simulink model "Model_Platform"  (R2018a)
settings: Solver=ode1  StartTime=0.0  StopTime=inf  FixedStep=0.001  RelTol=1e-3  EnableMultiTasking=on
PreLoadFcn:
  | ;HLABlocksetInit;;HLABlocksetInit;;HLABlocksetInit;
PostLoadFcn:
  | ;set_param(gcs,'PostCodeGenCommand', 'rtw_defines(buildInfo)');;set_param(gcs,'PostCodeGenCommand', 'rtw_defines(buildInfo)');;set_param(gcs,'PostCodeGenCommand', 'rtw_defines(buildInfo)');
undefined symbols (not defined in the file or in its folder): eng_speed, Heading_init, inertiaLateral, Joystick, Newton, omega_engine, omega_max, omega_wheel, Para, radiusWheel, Raphson, Standard_Devices, torque, Torque_lost, Torque_lost_wheel, X_init, Y_init, Z_init
libraries: simulink x26, dspnetwork x4, rtwinlib x2, PC_Simulator_Lib x2, vrlib x1
(part 4 of 4)

== system Model_Platform/Vehicle model/Drive_Train/4_Wheels_drive_train_and_Brake/FL/Alpha_Kappa_Selector2/alpha_calc/front ==
  Vy : Inport
  Vx : Inport  Port=2
  steering_angle : Inport  Port=3
  Constant : Constant  Value=0.001
  Divide : Product  Inputs=*/
  Fcn : Fcn  Expr=atan(u)
  Gain : Gain  Gain=180/pi
  Relational Operator : RelationalOperator  OutDataTypeStr=boolean  RndMeth=Nearest
  Subsystem1 : Subsystem
  Subtract : Sum  Inputs=+-
  Switch : Switch  Threshold=1
  alpha : Outport
  wires:
  Subsystem1/1(Out1) -> Divide/1
  Vx/1 -> Switch/1, Relational Operator/1
  Vy/1 -> Subsystem1/1(In1)
  Switch/1 -> Divide/2
  Fcn/1 -> Subtract/2
  Gain/1 -> alpha/1
  Divide/1 -> Fcn/1
  Subtract/1 -> Gain/1
  steering_angle/1 -> Subtract/1
  Constant/1 -> Relational Operator/2, Switch/3
  Relational Operator/1 -> Switch/2

== system Model_Platform/Vehicle model/Drive_Train/4_Wheels_drive_train_and_Brake/FR/Alpha_Kappa_Selector2/Dynamik Anteil2/Subsystem3 ==
  In1 : Inport
  Abs : Abs  SaturateOnIntegerOverflow=on
  In3_Switch : Constant
  Relational Operator : RelationalOperator  RndMeth=Nearest
  Switch : Switch  Threshold=1  SaturateOnIntegerOverflow=on
  Out1 : Outport
  wires:
  Switch/1 -> Out1/1
  Relational Operator/1 -> Switch/2
  In3_Switch/1 -> Switch/3, Relational Operator/2
  Abs/1 -> Relational Operator/1
  In1/1 -> Abs/1, Switch/1

== system Model_Platform/Vehicle model/Drive_Train/4_Wheels_drive_train_and_Brake/FR/Alpha_Kappa_Selector2/alpha_calc/Slip_angle_Calculation_From_Vx_and_Vy1 ==
  Vx_CoG[m|s] : Inport
  Vy_CoG[m|s] : Inport  Port=2
  Add : Sum
  Add2 : Sum
  Compare To Constant1 : simulink/Logic and Bit Operations/Compare To Constant  relop=>=  const=1  OutDataTypeStr=boolean
  Constant1 : Constant  Value=eps
  Data Type Conversion : DataTypeConversion
  Divide : Product  Inputs=*/
  Gain : Gain  Gain=180/pi
  Math Function : Math  Operator=square  SaturateOnIntegerOverflow=on
  Math Function1 : Math  Operator=square  SaturateOnIntegerOverflow=on
  Product1 : Product  Inputs=3
  Sign : Signum
  Sqrt : Sqrt  AlgorithmType=Newton-Raphson  SaturateOnIntegerOverflow=on
  Trigonometric Function1 : Trigonometry  Operator=atan
  Unary Minus1 : UnaryMinus
  Slip_Angle[deg] : Outport
  wires:
  Unary Minus1/1 -> Product1/3
  Sign/1 -> Unary Minus1/1
  Trigonometric Function1/1 -> Product1/1
  Constant1/1 -> Add2/2
  Add2/1 -> Divide/2
  Divide/1 -> Trigonometric Function1/1
  Sqrt/1 -> Compare To Constant1/1
  Add/1 -> Sqrt/1
  Math Function1/1 -> Add/2
  Math Function/1 -> Add/1
  Vx_CoG[m|s]/1 -> Add2/1, Math Function/1, Sign/1
  Vy_CoG[m|s]/1 -> Divide/1, Math Function1/1
  Compare To Constant1/1 -> Data Type Conversion/1
  Data Type Conversion/1 -> Product1/2
  Product1/1 -> Gain/1
  Gain/1 -> Slip_Angle[deg]/1

== system Model_Platform/Vehicle model/Drive_Train/4_Wheels_drive_train_and_Brake/FR/Alpha_Kappa_Selector2/alpha_calc/front ==
  Vy : Inport
  Vx : Inport  Port=2
  steering_angle : Inport  Port=3
  Constant : Constant  Value=0.001
  Divide : Product  Inputs=*/
  Fcn : Fcn  Expr=atan(u)
  Gain : Gain  Gain=180/pi
  Relational Operator : RelationalOperator  OutDataTypeStr=boolean  RndMeth=Nearest
  Subsystem1 : Subsystem
  Subtract : Sum  Inputs=+-
  Switch : Switch  Threshold=1
  alpha : Outport
  wires:
  Subsystem1/1(Out1) -> Divide/1
  Vx/1 -> Switch/1, Relational Operator/1
  Vy/1 -> Subsystem1/1(In1)
  Switch/1 -> Divide/2
  Fcn/1 -> Subtract/2
  Gain/1 -> alpha/1
  Divide/1 -> Fcn/1
  Subtract/1 -> Gain/1
  steering_angle/1 -> Subtract/1
  Constant/1 -> Relational Operator/2, Switch/3
  Relational Operator/1 -> Switch/2

== system Model_Platform/Vehicle model/Drive_Train/4_Wheels_drive_train_and_Brake/RL/Alpha_Kappa_Selector2/Dynamik Anteil2/Subsystem3 ==
  In1 : Inport
  Abs : Abs  SaturateOnIntegerOverflow=on
  In3_Switch : Constant
  Relational Operator : RelationalOperator  RndMeth=Nearest
  Switch : Switch  Threshold=1  SaturateOnIntegerOverflow=on
  Out1 : Outport
  wires:
  Switch/1 -> Out1/1
  Relational Operator/1 -> Switch/2
  In3_Switch/1 -> Switch/3, Relational Operator/2
  Abs/1 -> Relational Operator/1
  In1/1 -> Abs/1, Switch/1

== system Model_Platform/Vehicle model/Drive_Train/4_Wheels_drive_train_and_Brake/RL/Alpha_Kappa_Selector2/alpha_calc/Slip_angle_Calculation_From_Vx_and_Vy1 ==
  Vx_CoG[m|s] : Inport
  Vy_CoG[m|s] : Inport  Port=2
  Add : Sum
  Add2 : Sum
  Compare To Constant1 : simulink/Logic and Bit Operations/Compare To Constant  relop=>=  const=1  OutDataTypeStr=boolean
  Constant1 : Constant  Value=eps
  Data Type Conversion : DataTypeConversion
  Divide : Product  Inputs=*/
  Gain : Gain  Gain=180/pi
  Math Function : Math  Operator=square  SaturateOnIntegerOverflow=on
  Math Function1 : Math  Operator=square  SaturateOnIntegerOverflow=on
  Product1 : Product  Inputs=3
  Sign : Signum
  Sqrt : Sqrt  AlgorithmType=Newton-Raphson  SaturateOnIntegerOverflow=on
  Trigonometric Function1 : Trigonometry  Operator=atan
  Unary Minus1 : UnaryMinus
  Slip_Angle[deg] : Outport
  wires:
  Unary Minus1/1 -> Product1/3
  Sign/1 -> Unary Minus1/1
  Trigonometric Function1/1 -> Product1/1
  Constant1/1 -> Add2/2
  Add2/1 -> Divide/2
  Divide/1 -> Trigonometric Function1/1
  Sqrt/1 -> Compare To Constant1/1
  Add/1 -> Sqrt/1
  Math Function1/1 -> Add/2
  Math Function/1 -> Add/1
  Vx_CoG[m|s]/1 -> Add2/1, Math Function/1, Sign/1
  Vy_CoG[m|s]/1 -> Divide/1, Math Function1/1
  Compare To Constant1/1 -> Data Type Conversion/1
  Data Type Conversion/1 -> Product1/2
  Product1/1 -> Gain/1
  Gain/1 -> Slip_Angle[deg]/1

== system Model_Platform/Vehicle model/Drive_Train/4_Wheels_drive_train_and_Brake/RL/Alpha_Kappa_Selector2/alpha_calc/front ==
  Vy : Inport
  Vx : Inport  Port=2
  steering_angle : Inport  Port=3
  Constant : Constant  Value=0.001
  Divide : Product  Inputs=*/
  Fcn : Fcn  Expr=atan(u)
  Gain : Gain  Gain=180/pi
  Relational Operator : RelationalOperator  OutDataTypeStr=boolean  RndMeth=Nearest
  Subsystem1 : Subsystem
  Subtract : Sum  Inputs=+-
  Switch : Switch  Threshold=1
  alpha : Outport
  wires:
  Subsystem1/1(Out1) -> Divide/1
  Vx/1 -> Switch/1, Relational Operator/1
  Vy/1 -> Subsystem1/1(In1)
  Switch/1 -> Divide/2
  Fcn/1 -> Subtract/2
  Gain/1 -> alpha/1
  Divide/1 -> Fcn/1
  Subtract/1 -> Gain/1
  steering_angle/1 -> Subtract/1
  Constant/1 -> Relational Operator/2, Switch/3
  Relational Operator/1 -> Switch/2

== system Model_Platform/Vehicle model/Drive_Train/4_Wheels_drive_train_and_Brake/RR/Alpha_Kappa_Selector2/Dynamik Anteil2/Subsystem3 ==
  In1 : Inport
  Abs : Abs  SaturateOnIntegerOverflow=on
  In3_Switch : Constant
  Relational Operator : RelationalOperator  RndMeth=Nearest
  Switch : Switch  Threshold=1  SaturateOnIntegerOverflow=on
  Out1 : Outport
  wires:
  Switch/1 -> Out1/1
  Relational Operator/1 -> Switch/2
  In3_Switch/1 -> Switch/3, Relational Operator/2
  Abs/1 -> Relational Operator/1
  In1/1 -> Abs/1, Switch/1

== system Model_Platform/Vehicle model/Drive_Train/4_Wheels_drive_train_and_Brake/RR/Alpha_Kappa_Selector2/alpha_calc/Slip_angle_Calculation_From_Vx_and_Vy1 ==
  Vx_CoG[m|s] : Inport
  Vy_CoG[m|s] : Inport  Port=2
  Add : Sum
  Add2 : Sum
  Compare To Constant1 : simulink/Logic and Bit Operations/Compare To Constant  relop=>=  const=1  OutDataTypeStr=boolean
  Constant1 : Constant  Value=eps
  Data Type Conversion : DataTypeConversion
  Divide : Product  Inputs=*/
  Gain : Gain  Gain=180/pi
  Math Function : Math  Operator=square  SaturateOnIntegerOverflow=on
  Math Function1 : Math  Operator=square  SaturateOnIntegerOverflow=on
  Product1 : Product  Inputs=3
  Sign : Signum
  Sqrt : Sqrt  AlgorithmType=Newton-Raphson  SaturateOnIntegerOverflow=on
  Trigonometric Function1 : Trigonometry  Operator=atan
  Unary Minus1 : UnaryMinus
  Slip_Angle[deg] : Outport
  wires:
  Unary Minus1/1 -> Product1/3
  Sign/1 -> Unary Minus1/1
  Trigonometric Function1/1 -> Product1/1
  Constant1/1 -> Add2/2
  Add2/1 -> Divide/2
  Divide/1 -> Trigonometric Function1/1
  Sqrt/1 -> Compare To Constant1/1
  Add/1 -> Sqrt/1
  Math Function1/1 -> Add/2
  Math Function/1 -> Add/1
  Vx_CoG[m|s]/1 -> Add2/1, Math Function/1, Sign/1
  Vy_CoG[m|s]/1 -> Divide/1, Math Function1/1
  Compare To Constant1/1 -> Data Type Conversion/1
  Data Type Conversion/1 -> Product1/2
  Product1/1 -> Gain/1
  Gain/1 -> Slip_Angle[deg]/1

== system Model_Platform/Vehicle model/Drive_Train/4_Wheels_drive_train_and_Brake/RR/Alpha_Kappa_Selector2/alpha_calc/front ==
  Vy : Inport
  Vx : Inport  Port=2
  steering_angle : Inport  Port=3
  Constant : Constant  Value=0.001
  Divide : Product  Inputs=*/
  Fcn : Fcn  Expr=atan(u)
  Gain : Gain  Gain=180/pi
  Relational Operator : RelationalOperator  OutDataTypeStr=boolean  RndMeth=Nearest
  Subsystem1 : Subsystem
  Subtract : Sum  Inputs=+-
  Switch : Switch  Threshold=1
  alpha : Outport
  wires:
  Subsystem1/1(Out1) -> Divide/1
  Vx/1 -> Switch/1, Relational Operator/1
  Vy/1 -> Subsystem1/1(In1)
  Switch/1 -> Divide/2
  Fcn/1 -> Subtract/2
  Gain/1 -> alpha/1
  Divide/1 -> Fcn/1
  Subtract/1 -> Gain/1
  steering_angle/1 -> Subtract/1
  Constant/1 -> Relational Operator/2, Switch/3
  Relational Operator/1 -> Switch/2

== system Model_Platform/Vehicle model/Drive_Train/4_Wheels_drive_train_and_Brake/FL/Alpha_Kappa_Selector2/alpha_calc/front/Subsystem1 ==
  In1 : Inport
  Abs : Abs
  Constant1 : Constant  Value=0.005
  Constant2 : Constant  Value=0
  Relational Operator1 : RelationalOperator  OutDataTypeStr=boolean  RndMeth=Nearest
  Switch1 : Switch  Threshold=1
  Out1 : Outport
  wires:
  In1/1 -> Switch1/1, Abs/1
  Relational Operator1/1 -> Switch1/2
  Switch1/1 -> Out1/1
  Constant1/1 -> Relational Operator1/2
  Constant2/1 -> Switch1/3
  Abs/1 -> Relational Operator1/1

== system Model_Platform/Vehicle model/Drive_Train/4_Wheels_drive_train_and_Brake/FR/Alpha_Kappa_Selector2/alpha_calc/front/Subsystem1 ==
  In1 : Inport
  Abs : Abs
  Constant1 : Constant  Value=0.005
  Constant2 : Constant  Value=0
  Relational Operator1 : RelationalOperator  OutDataTypeStr=boolean  RndMeth=Nearest
  Switch1 : Switch  Threshold=1
  Out1 : Outport
  wires:
  In1/1 -> Switch1/1, Abs/1
  Relational Operator1/1 -> Switch1/2
  Switch1/1 -> Out1/1
  Constant1/1 -> Relational Operator1/2
  Constant2/1 -> Switch1/3
  Abs/1 -> Relational Operator1/1

== system Model_Platform/Vehicle model/Drive_Train/4_Wheels_drive_train_and_Brake/RL/Alpha_Kappa_Selector2/alpha_calc/front/Subsystem1 ==
  In1 : Inport
  Abs : Abs
  Constant1 : Constant  Value=0.005
  Constant2 : Constant  Value=0
  Relational Operator1 : RelationalOperator  OutDataTypeStr=boolean  RndMeth=Nearest
  Switch1 : Switch  Threshold=1
  Out1 : Outport
  wires:
  In1/1 -> Switch1/1, Abs/1
  Relational Operator1/1 -> Switch1/2
  Switch1/1 -> Out1/1
  Constant1/1 -> Relational Operator1/2
  Constant2/1 -> Switch1/3
  Abs/1 -> Relational Operator1/1

== system Model_Platform/Vehicle model/Drive_Train/4_Wheels_drive_train_and_Brake/RR/Alpha_Kappa_Selector2/alpha_calc/front/Subsystem1 ==
  In1 : Inport
  Abs : Abs
  Constant1 : Constant  Value=0.005
  Constant2 : Constant  Value=0
  Relational Operator1 : RelationalOperator  OutDataTypeStr=boolean  RndMeth=Nearest
  Switch1 : Switch  Threshold=1
  Out1 : Outport
  wires:
  In1/1 -> Switch1/1, Abs/1
  Relational Operator1/1 -> Switch1/2
  Switch1/1 -> Out1/1
  Constant1/1 -> Relational Operator1/2
  Constant2/1 -> Switch1/3
  Abs/1 -> Relational Operator1/1

== matlab function Model_Platform/Vehicle model/Drive_Train/4_Wheels_drive_train_and_Brake/FL/Fx_calculator ==
  data: lambda input; Fx output; alpha input; Fz input; mue input
 function Fx = FM_Fx(lambda,alpha,Fz,mue)
% This block supports an embeddable subset of the MATLAB language.
% See the help menu for details. 

%% Längstkraft
kappa=lambda;
a=tan(alpha*pi/180);
F_z=Fz;
% Parameter
p_Cx1=1.685;
p_Ex1=0.344;
p_Ex2=0.095;
p_Ex3=-0.02;
p_Ex4=0;
p_Kx1=21.51;
p_Kx2=-0.163;
p_Kx3=0.245;
p_Hx1=0;
p_Hx2=0;
p_Vx1=0;
p_Vx2=0;
r_Cx1=1.0902;
r_Bx1=12.35;
r_Bx2=-10.77;
r_Bx3=0;
r_Ex1=0;
r_Ex2=0;
r_Hx1=0.007;            %r_Hx1=0.007;
gamma=0;
lambda_xa=1;
lambda_Cx=1;
lambda_Ex=1;
lambda_Hx=1;
lambda_Vx=1;
lambda_Kxkappa=1;
% Unter der Annahme, dass die Vertikallast unverändert bleibt:
df_z=0;

%F_z=5500;
%mue=0.7;
chi_1=1;

% Berechnung:

B_xa=(r_Bx1+r_Bx3*gamma^2)*cos(atan(r_Bx2*kappa))*lambda_xa;
C_xa=r_Cx1;
E_xa=r_Ex1+r_Ex2*df_z;

S_Hxa=r_Hx1;
a_S=a+S_Hxa;

G_xa0=cos(C_xa*atan(B_xa*S_Hxa-E_xa*(B_xa*S_Hxa-atan(B_xa*S_Hxa))));
G_xa=cos(C_xa*atan(B_xa*a_S-E_xa*(B_xa*a_S-atan(B_xa*a_S))))/G_xa0;

K_xkappa=F_z*(p_Kx1+p_Kx2*df_z)*exp(p_Kx3*df_z)*lambda_Kxkappa;
C_x=p_Cx1*lambda_Cx;
D_x=mue*F_z*chi_1;
B_x=K_xkappa/(C_x*D_x+eps);
E_x=(p_Ex1+p_Ex2*df_z+p_Ex3*df_z^2)*(1-p_Ex4*sign(kappa))*lambda_Ex;

S_Vx=F_z*(p_Vx1+p_Vx2*df_z)*lambda_Vx*lambda_Hx*chi_1;
S_Hx=(p_Hx1+p_Hx2*df_z)*lambda_Hx;
kappa_x=kappa+S_Hx;

F_x0 = D_x*sin(C_x*atan(B_x*kappa_x-E_x*(B_x*kappa_x-atan(B_x*kappa_x))))+S_Vx;
% F_x0 = D_x*sin(C_x*atan(B_x*kappa_x-E_x.*(B_x*kappa_x-atan(B_x*kappa_x))))+S_Vx;
F_x = G_xa*F_x0;
% if F_x>249;
%     F_x=249;
% end
Fx=F_x;

== stateflow chart Model_Platform/Vehicle model/Drive_Train/Gearbox/Automatic_Gear_box_Controller ==
  state fourth
    entry: gear=4;
  state second
    entry: gear=2;
  state third
    entry: gear=3;
  state fifth
    entry: gear=5;
  state first
    entry: gear=1;
  state neutral
    entry: gear=0;
  state reverse
    entry: gear= 6;
  second -> third [order 2] : [velocity>30&& omega>4000]
  third -> fourth [order 2] : [velocity>60&& omega>4000]
  (default) -> neutral
  first -> second [order 1] : [velocity>10&& omega>4000]
  fourth -> fifth [order 3] : [velocity>90&& omega>4000]
  reverse -> neutral : [DNR==1]
  neutral -> first [order 1] : [DNR==1]
  second -> neutral [order 3] : [DNR==0]
  second -> first [order 1] : [velocity<5]
  third -> second [order 1] : [velocity<30]
  third -> neutral [order 3] : [DNR==0]
  fourth -> third [order 1] : [velocity<50]
  first -> neutral [order 2] : [DNR==-1]
  fourth -> neutral [order 2] : [DNR==0]
  fifth -> fourth [order 1] : [velocity<80]
  fifth -> neutral [order 2] : [DNR==0]
  neutral -> reverse [order 2] : [DNR==-1&& velocity<1]
  data: velocity input; DNR input; gear output double; omega input

== matlab function Model_Platform/Vehicle model/Drive_Train/4_Wheels_drive_train_and_Brake/FL/Fy_calculator ==
  data: lambda input; Fy output; alpha input; V_x input; Fz input; mue input

function Fy = FM_Fy(lambda,alpha,V_x,Fz,mue)
% This block supports an embeddable subset of the MATLAB language.
% See the help menu for details. 
%% Querkraft

kappa=lambda;
a=tan(alpha*pi/180);
%if V_x >=0 
 %   sign=1;
%else
 %   sign=-1;
%end
a_star=tan(alpha*pi/180)*sign(V_x);
F_z=Fz;
%Parameter

p_Cy1=1.193;
p_Ey1=-1.003;
p_Ey2=-0.532;
p_Ey3=-0.083;
p_Ey4=-4.787;
p_Ey5=0;
p_Ky1=14.95;
p_Ky2=2.13;
p_Ky3=-0.028;
p_Ky4=2;
p_Ky5=0;
p_Ky6=2.5;
p_Ky7=0;
p_Hy1=0;
p_Hy2=0;
p_Vy1=0;
p_Vy2=0;
p_Vy3=0;
p_Vy4=0;
r_By1=6.461;
r_By2=4.196;
r_By3=-0.015;
r_Cy1=1.081;
r_Ey1=0;
r_Ey2=0;
r_Hy1=0;
r_Hy2=0;
r_Vy1=0;
r_Vy2=0;
r_Vy3=0;
r_Vy4=0;
r_Vy5=0;
r_Vy6=0;

lambda_ykappa=1;
lambda_Fz0=1;
lambda_Kya=1;
lambda_Cy=1;
lambda_Vy=1;
lambda_muey=1;
lambda_Hy=1;
lambda_Kygamma=1;
lambda_Ey=1;
lambda_Vykappa=1;

% Unter der Annahme, dass die Vertikallast unverändert bleibt:
df_z=0;

%F_z=5500;
%mue=0.7;
chi_0=1;
chi_1=1;
chi_2=1;
chi_3=1;
chi_4=1;

% Annamhe, dass der Sturz bei null bleibt;

gamma=0;

% Berechnung

B_ykappa=(r_By1+r_By3*gamma^2)*cos(atan(r_By2*(a_star-r_By3)))*lambda_ykappa;
C_ykappa=r_Cy1;
E_ykappa=r_Ey1+r_Ey2*df_z;

S_Hykappa=r_Hy1+r_Hy2*df_z;
kappa_S=kappa+S_Hykappa;

G_ykappa0=cos(C_ykappa*atan(B_ykappa*S_Hykappa-E_ykappa*(B_ykappa*S_Hykappa-atan(B_ykappa*S_Hykappa))));
G_ykappa=cos(C_ykappa*atan(B_ykappa*kappa_S-E_ykappa*(B_ykappa*kappa_S-atan(B_ykappa*kappa_S))))/G_ykappa0;
% G_ykappa=cos(C_ykappa*atan(B_ykappa.*kappa_S-E_ykappa*(B_ykappa.*kappa_S-atan(B_ykappa.*kappa_S))))/G_ykappa0;















K_ygamma0=F_z*(p_Ky6+p_Ky7*df_z)*lambda_Kygamma;
S_Vygamma=F_z*(p_Vy3+p_Vy4*df_z)*gamma*lambda_Kygamma*lambda_muey*chi_2;
K_ya=p_Ky1*lambda_Fz0*F_z*sin(p_Ky4*atan(F_z/((p_Ky2+p_Ky5*gamma^2)*lambda_Fz0*F_z)))/(1+p_Ky3*gamma^2)*chi_3*lambda_Kya;
S_Vy=F_z*(p_Vy1+p_Vy2*df_z)*lambda_Vy*lambda_muey*chi_2+S_Vygamma;
S_Hy=(p_Hy1+p_Hy2*df_z)*lambda_Hy+(K_ygamma0*gamma-S_Vygamma)*chi_0/(K_ya+eps)+chi_4-1;

a_y=a+S_Hy;

D_Vykappa=mue*F_z*(r_Vy1+r_Vy2*df_z+r_Vy3*gamma)*cos(atan(r_Vy4*a))*chi_2;
S_Vykappa=D_Vykappa*sin(r_Vy5*atan(r_Vy6*kappa))*lambda_Vykappa;

C_y=p_Cy1*lambda_Cy;
D_y=mue*F_z*chi_2;
B_y=K_ya/(C_y*D_y+eps);
E_y=(p_Ey1+p_Ey2*df_z)*(1+p_Ey5*gamma^2-(p_Ey3+p_Ey4*gamma)*sign(a_y))*lambda_Ey;

F_y0=D_y*sin(C_y*atan(B_y*a_y-E_y*(B_y*a_y-atan(B_y*a_y))))+S_Vy;

F_y=G_ykappa*F_y0+S_Vykappa;

Fy=F_y;

== matlab function Model_Platform/Vehicle model/HMI_Realtime_normal_mode/HMI_Logitech1/MATLAB Function ==
  data: accPedal input; brake output; brakePedal input
function brake = fcn(accPedal,brakePedal)
%#codegen

if (accPedal  >= 0.99 && brakePedal >= 0.99) % No acc & No brake 
        brake = 0.8;                         % Apply slight brake
elseif (accPedal <= 0.99)                        % Acc press
        brake = 1;                           % No brake
else 
        brake = brakePedal;
end

== matlab function Model_Platform/Vehicle model/Drive_Train/4_Wheels_drive_train_and_Brake/RL/Fx_calculator ==
  data: lambda input; Fx output; alpha input; Fz input; mue input
 function Fx = FM_Fx(lambda,alpha,Fz,mue)
% This block supports an embeddable subset of the MATLAB language.
% See the help menu for details. 

%% Längstkraft
kappa=lambda;
a=tan(alpha*pi/180);
F_z=Fz;
% Parameter
p_Cx1=1.685;
p_Ex1=0.344;
p_Ex2=0.095;
p_Ex3=-0.02;
p_Ex4=0;
p_Kx1=21.51;
p_Kx2=-0.163;
p_Kx3=0.245;
p_Hx1=0;
p_Hx2=0;
p_Vx1=0;
p_Vx2=0;
r_Cx1=1.0902;
r_Bx1=12.35;
r_Bx2=-10.77;
r_Bx3=0;
r_Ex1=0;
r_Ex2=0;
r_Hx1=0.007;            %r_Hx1=0.007;
gamma=0;
lambda_xa=1;
lambda_Cx=1;
lambda_Ex=1;
lambda_Hx=1;
lambda_Vx=1;
lambda_Kxkappa=1;
% Unter der Annahme, dass die Vertikallast unverändert bleibt:
df_z=0;

%F_z=5500;
%mue=0.7;
chi_1=1;

% Berechnung:

B_xa=(r_Bx1+r_Bx3*gamma^2)*cos(atan(r_Bx2*kappa))*lambda_xa;
C_xa=r_Cx1;
E_xa=r_Ex1+r_Ex2*df_z;

S_Hxa=r_Hx1;
a_S=a+S_Hxa;

G_xa0=cos(C_xa*atan(B_xa*S_Hxa-E_xa*(B_xa*S_Hxa-atan(B_xa*S_Hxa))));
G_xa=cos(C_xa*atan(B_xa*a_S-E_xa*(B_xa*a_S-atan(B_xa*a_S))))/G_xa0;

K_xkappa=F_z*(p_Kx1+p_Kx2*df_z)*exp(p_Kx3*df_z)*lambda_Kxkappa;
C_x=p_Cx1*lambda_Cx;
D_x=mue*F_z*chi_1;
B_x=K_xkappa/(C_x*D_x+eps);
E_x=(p_Ex1+p_Ex2*df_z+p_Ex3*df_z^2)*(1-p_Ex4*sign(kappa))*lambda_Ex;

S_Vx=F_z*(p_Vx1+p_Vx2*df_z)*lambda_Vx*lambda_Hx*chi_1;
S_Hx=(p_Hx1+p_Hx2*df_z)*lambda_Hx;
kappa_x=kappa+S_Hx;

F_x0 = D_x*sin(C_x*atan(B_x*kappa_x-E_x*(B_x*kappa_x-atan(B_x*kappa_x))))+S_Vx;
% F_x0 = D_x*sin(C_x*atan(B_x*kappa_x-E_x.*(B_x*kappa_x-atan(B_x*kappa_x))))+S_Vx;
F_x = G_xa*F_x0;
% if F_x>249;
%     F_x=249;
% end
Fx=F_x;

== matlab function Model_Platform/Vehicle model/Drive_Train/4_Wheels_drive_train_and_Brake/RL/Fy_calculator ==
  data: lambda input; Fy output; alpha input; V_x input; Fz input; mue input

function Fy = FM_Fy(lambda,alpha,V_x,Fz,mue)
% This block supports an embeddable subset of the MATLAB language.
% See the help menu for details. 
%% Querkraft

kappa=lambda;
a=tan(alpha*pi/180);
%if V_x >=0 
 %   sign=1;
%else
 %   sign=-1;
%end
a_star=tan(alpha*pi/180)*sign(V_x);
F_z=Fz;
%Parameter

p_Cy1=1.193;
p_Ey1=-1.003;
p_Ey2=-0.532;
p_Ey3=-0.083;
p_Ey4=-4.787;
p_Ey5=0;
p_Ky1=14.95;
p_Ky2=2.13;
p_Ky3=-0.028;
p_Ky4=2;
p_Ky5=0;
p_Ky6=2.5;
p_Ky7=0;
p_Hy1=0;
p_Hy2=0;
p_Vy1=0;
p_Vy2=0;
p_Vy3=0;
p_Vy4=0;
r_By1=6.461;
r_By2=4.196;
r_By3=-0.015;
r_Cy1=1.081;
r_Ey1=0;
r_Ey2=0;
r_Hy1=0;
r_Hy2=0;
r_Vy1=0;
r_Vy2=0;
r_Vy3=0;
r_Vy4=0;
r_Vy5=0;
r_Vy6=0;

lambda_ykappa=1;
lambda_Fz0=1;
lambda_Kya=1;
lambda_Cy=1;
lambda_Vy=1;
lambda_muey=1;
lambda_Hy=1;
lambda_Kygamma=1;
lambda_Ey=1;
lambda_Vykappa=1;

% Unter der Annahme, dass die Vertikallast unverändert bleibt:
df_z=0;

%F_z=5500;
%mue=0.7;
chi_0=1;
chi_1=1;
chi_2=1;
chi_3=1;
chi_4=1;

% Annamhe, dass der Sturz bei null bleibt;

gamma=0;

% Berechnung

B_ykappa=(r_By1+r_By3*gamma^2)*cos(atan(r_By2*(a_star-r_By3)))*lambda_ykappa;
C_ykappa=r_Cy1;
E_ykappa=r_Ey1+r_Ey2*df_z;

S_Hykappa=r_Hy1+r_Hy2*df_z;
kappa_S=kappa+S_Hykappa;

G_ykappa0=cos(C_ykappa*atan(B_ykappa*S_Hykappa-E_ykappa*(B_ykappa*S_Hykappa-atan(B_ykappa*S_Hykappa))));
G_ykappa=cos(C_ykappa*atan(B_ykappa*kappa_S-E_ykappa*(B_ykappa*kappa_S-atan(B_ykappa*kappa_S))))/G_ykappa0;
% G_ykappa=cos(C_ykappa*atan(B_ykappa.*kappa_S-E_ykappa*(B_ykappa.*kappa_S-atan(B_ykappa.*kappa_S))))/G_ykappa0;















K_ygamma0=F_z*(p_Ky6+p_Ky7*df_z)*lambda_Kygamma;
S_Vygamma=F_z*(p_Vy3+p_Vy4*df_z)*gamma*lambda_Kygamma*lambda_muey*chi_2;
K_ya=p_Ky1*lambda_Fz0*F_z*sin(p_Ky4*atan(F_z/((p_Ky2+p_Ky5*gamma^2)*lambda_Fz0*F_z)))/(1+p_Ky3*gamma^2)*chi_3*lambda_Kya;
S_Vy=F_z*(p_Vy1+p_Vy2*df_z)*lambda_Vy*lambda_muey*chi_2+S_Vygamma;
S_Hy=(p_Hy1+p_Hy2*df_z)*lambda_Hy+(K_ygamma0*gamma-S_Vygamma)*chi_0/(K_ya+eps)+chi_4-1;

a_y=a+S_Hy;

D_Vykappa=mue*F_z*(r_Vy1+r_Vy2*df_z+r_Vy3*gamma)*cos(atan(r_Vy4*a))*chi_2;
S_Vykappa=D_Vykappa*sin(r_Vy5*atan(r_Vy6*kappa))*lambda_Vykappa;

C_y=p_Cy1*lambda_Cy;
D_y=mue*F_z*chi_2;
B_y=K_ya/(C_y*D_y+eps);
E_y=(p_Ey1+p_Ey2*df_z)*(1+p_Ey5*gamma^2-(p_Ey3+p_Ey4*gamma)*sign(a_y))*lambda_Ey;

F_y0=D_y*sin(C_y*atan(B_y*a_y-E_y*(B_y*a_y-atan(B_y*a_y))))+S_Vy;

F_y=G_ykappa*F_y0+S_Vykappa;

Fy=F_y;

== matlab function Model_Platform/Vehicle model/Drive_Train/4_Wheels_drive_train_and_Brake/RR/Fx_calculator ==
  data: lambda input; Fx output; alpha input; Fz input; mue input
 function Fx = FM_Fx(lambda,alpha,Fz,mue)
% This block supports an embeddable subset of the MATLAB language.
% See the help menu for details. 

%% Längstkraft
kappa=lambda;
a=tan(alpha*pi/180);
F_z=Fz;
% Parameter
p_Cx1=1.685;
p_Ex1=0.344;
p_Ex2=0.095;
p_Ex3=-0.02;
p_Ex4=0;
p_Kx1=21.51;
p_Kx2=-0.163;
p_Kx3=0.245;
p_Hx1=0;
p_Hx2=0;
p_Vx1=0;
p_Vx2=0;
r_Cx1=1.0902;
r_Bx1=12.35;
r_Bx2=-10.77;
r_Bx3=0;
r_Ex1=0;
r_Ex2=0;
r_Hx1=0.007;            %r_Hx1=0.007;
gamma=0;
lambda_xa=1;
lambda_Cx=1;
lambda_Ex=1;
lambda_Hx=1;
lambda_Vx=1;
lambda_Kxkappa=1;
% Unter der Annahme, dass die Vertikallast unverändert bleibt:
df_z=0;

%F_z=5500;
%mue=0.7;
chi_1=1;

% Berechnung:

B_xa=(r_Bx1+r_Bx3*gamma^2)*cos(atan(r_Bx2*kappa))*lambda_xa;
C_xa=r_Cx1;
E_xa=r_Ex1+r_Ex2*df_z;

S_Hxa=r_Hx1;
a_S=a+S_Hxa;

G_xa0=cos(C_xa*atan(B_xa*S_Hxa-E_xa*(B_xa*S_Hxa-atan(B_xa*S_Hxa))));
G_xa=cos(C_xa*atan(B_xa*a_S-E_xa*(B_xa*a_S-atan(B_xa*a_S))))/G_xa0;

K_xkappa=F_z*(p_Kx1+p_Kx2*df_z)*exp(p_Kx3*df_z)*lambda_Kxkappa;
C_x=p_Cx1*lambda_Cx;
D_x=mue*F_z*chi_1;
B_x=K_xkappa/(C_x*D_x+eps);
E_x=(p_Ex1+p_Ex2*df_z+p_Ex3*df_z^2)*(1-p_Ex4*sign(kappa))*lambda_Ex;

S_Vx=F_z*(p_Vx1+p_Vx2*df_z)*lambda_Vx*lambda_Hx*chi_1;
S_Hx=(p_Hx1+p_Hx2*df_z)*lambda_Hx;
kappa_x=kappa+S_Hx;

F_x0 = D_x*sin(C_x*atan(B_x*kappa_x-E_x*(B_x*kappa_x-atan(B_x*kappa_x))))+S_Vx;
% F_x0 = D_x*sin(C_x*atan(B_x*kappa_x-E_x.*(B_x*kappa_x-atan(B_x*kappa_x))))+S_Vx;
F_x = G_xa*F_x0;
% if F_x>249;
%     F_x=249;
% end
Fx=F_x;

== matlab function Model_Platform/Vehicle model/Drive_Train/4_Wheels_drive_train_and_Brake/RR/Fy_calculator ==
  data: lambda input; Fy output; alpha input; V_x input; Fz input; mue input

function Fy = FM_Fy(lambda,alpha,V_x,Fz,mue)
% This block supports an embeddable subset of the MATLAB language.
% See the help menu for details. 
%% Querkraft

kappa=lambda;
a=tan(alpha*pi/180);
%if V_x >=0 
 %   sign=1;
%else
 %   sign=-1;
%end
a_star=tan(alpha*pi/180)*sign(V_x);
F_z=Fz;
%Parameter

p_Cy1=1.193;
p_Ey1=-1.003;
p_Ey2=-0.532;
p_Ey3=-0.083;
p_Ey4=-4.787;
p_Ey5=0;
p_Ky1=14.95;
p_Ky2=2.13;
p_Ky3=-0.028;
p_Ky4=2;
p_Ky5=0;
p_Ky6=2.5;
p_Ky7=0;
p_Hy1=0;
p_Hy2=0;
p_Vy1=0;
p_Vy2=0;
p_Vy3=0;
p_Vy4=0;
r_By1=6.461;
r_By2=4.196;
r_By3=-0.015;
r_Cy1=1.081;
r_Ey1=0;
r_Ey2=0;
r_Hy1=0;
r_Hy2=0;
r_Vy1=0;
r_Vy2=0;
r_Vy3=0;
r_Vy4=0;
r_Vy5=0;
r_Vy6=0;

lambda_ykappa=1;
lambda_Fz0=1;
lambda_Kya=1;
lambda_Cy=1;
lambda_Vy=1;
lambda_muey=1;
lambda_Hy=1;
lambda_Kygamma=1;
lambda_Ey=1;
lambda_Vykappa=1;

% Unter der Annahme, dass die Vertikallast unverändert bleibt:
df_z=0;

%F_z=5500;
%mue=0.7;
chi_0=1;
chi_1=1;
chi_2=1;
chi_3=1;
chi_4=1;

% Annamhe, dass der Sturz bei null bleibt;

gamma=0;

% Berechnung

B_ykappa=(r_By1+r_By3*gamma^2)*cos(atan(r_By2*(a_star-r_By3)))*lambda_ykappa;
C_ykappa=r_Cy1;
E_ykappa=r_Ey1+r_Ey2*df_z;

S_Hykappa=r_Hy1+r_Hy2*df_z;
kappa_S=kappa+S_Hykappa;

G_ykappa0=cos(C_ykappa*atan(B_ykappa*S_Hykappa-E_ykappa*(B_ykappa*S_Hykappa-atan(B_ykappa*S_Hykappa))));
G_ykappa=cos(C_ykappa*atan(B_ykappa*kappa_S-E_ykappa*(B_ykappa*kappa_S-atan(B_ykappa*kappa_S))))/G_ykappa0;
% G_ykappa=cos(C_ykappa*atan(B_ykappa.*kappa_S-E_ykappa*(B_ykappa.*kappa_S-atan(B_ykappa.*kappa_S))))/G_ykappa0;















K_ygamma0=F_z*(p_Ky6+p_Ky7*df_z)*lambda_Kygamma;
S_Vygamma=F_z*(p_Vy3+p_Vy4*df_z)*gamma*lambda_Kygamma*lambda_muey*chi_2;
K_ya=p_Ky1*lambda_Fz0*F_z*sin(p_Ky4*atan(F_z/((p_Ky2+p_Ky5*gamma^2)*lambda_Fz0*F_z)))/(1+p_Ky3*gamma^2)*chi_3*lambda_Kya;
S_Vy=F_z*(p_Vy1+p_Vy2*df_z)*lambda_Vy*lambda_muey*chi_2+S_Vygamma;
S_Hy=(p_Hy1+p_Hy2*df_z)*lambda_Hy+(K_ygamma0*gamma-S_Vygamma)*chi_0/(K_ya+eps)+chi_4-1;

a_y=a+S_Hy;

D_Vykappa=mue*F_z*(r_Vy1+r_Vy2*df_z+r_Vy3*gamma)*cos(atan(r_Vy4*a))*chi_2;
S_Vykappa=D_Vykappa*sin(r_Vy5*atan(r_Vy6*kappa))*lambda_Vykappa;

C_y=p_Cy1*lambda_Cy;
D_y=mue*F_z*chi_2;
B_y=K_ya/(C_y*D_y+eps);
E_y=(p_Ey1+p_Ey2*df_z)*(1+p_Ey5*gamma^2-(p_Ey3+p_Ey4*gamma)*sign(a_y))*lambda_Ey;

F_y0=D_y*sin(C_y*atan(B_y*a_y-E_y*(B_y*a_y-atan(B_y*a_y))))+S_Vy;

F_y=G_ykappa*F_y0+S_Vykappa;

Fy=F_y;

== matlab function Model_Platform/Vehicle model/Drive_Train/4_Wheels_drive_train_and_Brake/FR/Fx_calculator ==
  data: lambda input; Fx output; alpha input; Fz input; mue input
 function Fx = FM_Fx(lambda,alpha,Fz,mue)
% This block supports an embeddable subset of the MATLAB language.
% See the help menu for details. 

%% Längstkraft
kappa=lambda;
a=tan(alpha*pi/180);
F_z=Fz;
% Parameter
p_Cx1=1.685;
p_Ex1=0.344;
p_Ex2=0.095;
p_Ex3=-0.02;
p_Ex4=0;
p_Kx1=21.51;
p_Kx2=-0.163;
p_Kx3=0.245;
p_Hx1=0;
p_Hx2=0;
p_Vx1=0;
p_Vx2=0;
r_Cx1=1.0902;
r_Bx1=12.35;
r_Bx2=-10.77;
r_Bx3=0;
r_Ex1=0;
r_Ex2=0;
r_Hx1=0.007;            %r_Hx1=0.007;
gamma=0;
lambda_xa=1;
lambda_Cx=1;
lambda_Ex=1;
lambda_Hx=1;
lambda_Vx=1;
lambda_Kxkappa=1;
% Unter der Annahme, dass die Vertikallast unverändert bleibt:
df_z=0;

%F_z=5500;
%mue=0.7;
chi_1=1;

% Berechnung:

B_xa=(r_Bx1+r_Bx3*gamma^2)*cos(atan(r_Bx2*kappa))*lambda_xa;
C_xa=r_Cx1;
E_xa=r_Ex1+r_Ex2*df_z;

S_Hxa=r_Hx1;
a_S=a+S_Hxa;

G_xa0=cos(C_xa*atan(B_xa*S_Hxa-E_xa*(B_xa*S_Hxa-atan(B_xa*S_Hxa))));
G_xa=cos(C_xa*atan(B_xa*a_S-E_xa*(B_xa*a_S-atan(B_xa*a_S))))/G_xa0;

K_xkappa=F_z*(p_Kx1+p_Kx2*df_z)*exp(p_Kx3*df_z)*lambda_Kxkappa;
C_x=p_Cx1*lambda_Cx;
D_x=mue*F_z*chi_1;
B_x=K_xkappa/(C_x*D_x+eps);
E_x=(p_Ex1+p_Ex2*df_z+p_Ex3*df_z^2)*(1-p_Ex4*sign(kappa))*lambda_Ex;

S_Vx=F_z*(p_Vx1+p_Vx2*df_z)*lambda_Vx*lambda_Hx*chi_1;
S_Hx=(p_Hx1+p_Hx2*df_z)*lambda_Hx;
kappa_x=kappa+S_Hx;

F_x0 = D_x*sin(C_x*atan(B_x*kappa_x-E_x*(B_x*kappa_x-atan(B_x*kappa_x))))+S_Vx;
% F_x0 = D_x*sin(C_x*atan(B_x*kappa_x-E_x.*(B_x*kappa_x-atan(B_x*kappa_x))))+S_Vx;
F_x = G_xa*F_x0;
% if F_x>249;
%     F_x=249;
% end
Fx=F_x;

== matlab function Model_Platform/Vehicle model/Drive_Train/4_Wheels_drive_train_and_Brake/FR/Fy_calculator ==
  data: lambda input; Fy output; alpha input; V_x input; Fz input; mue input

function Fy = FM_Fy(lambda,alpha,V_x,Fz,mue)
% This block supports an embeddable subset of the MATLAB language.
% See the help menu for details. 
%% Querkraft

kappa=lambda;
a=tan(alpha*pi/180);
%if V_x >=0 
 %   sign=1;
%else
 %   sign=-1;
%end
a_star=tan(alpha*pi/180)*sign(V_x);
F_z=Fz;
%Parameter

p_Cy1=1.193;
p_Ey1=-1.003;
p_Ey2=-0.532;
p_Ey3=-0.083;
p_Ey4=-4.787;
p_Ey5=0;
p_Ky1=14.95;
p_Ky2=2.13;
p_Ky3=-0.028;
p_Ky4=2;
p_Ky5=0;
p_Ky6=2.5;
p_Ky7=0;
p_Hy1=0;
p_Hy2=0;
p_Vy1=0;
p_Vy2=0;
p_Vy3=0;
p_Vy4=0;
r_By1=6.461;
r_By2=4.196;
r_By3=-0.015;
r_Cy1=1.081;
r_Ey1=0;
r_Ey2=0;
r_Hy1=0;
r_Hy2=0;
r_Vy1=0;
r_Vy2=0;
r_Vy3=0;
r_Vy4=0;
r_Vy5=0;
r_Vy6=0;

lambda_ykappa=1;
lambda_Fz0=1;
lambda_Kya=1;
lambda_Cy=1;
lambda_Vy=1;
lambda_muey=1;
lambda_Hy=1;
lambda_Kygamma=1;
lambda_Ey=1;
lambda_Vykappa=1;

% Unter der Annahme, dass die Vertikallast unverändert bleibt:
df_z=0;

%F_z=5500;
%mue=0.7;
chi_0=1;
chi_1=1;
chi_2=1;
chi_3=1;
chi_4=1;

% Annamhe, dass der Sturz bei null bleibt;

gamma=0;

% Berechnung

B_ykappa=(r_By1+r_By3*gamma^2)*cos(atan(r_By2*(a_star-r_By3)))*lambda_ykappa;
C_ykappa=r_Cy1;
E_ykappa=r_Ey1+r_Ey2*df_z;

S_Hykappa=r_Hy1+r_Hy2*df_z;
kappa_S=kappa+S_Hykappa;

G_ykappa0=cos(C_ykappa*atan(B_ykappa*S_Hykappa-E_ykappa*(B_ykappa*S_Hykappa-atan(B_ykappa*S_Hykappa))));
G_ykappa=cos(C_ykappa*atan(B_ykappa*kappa_S-E_ykappa*(B_ykappa*kappa_S-atan(B_ykappa*kappa_S))))/G_ykappa0;
% G_ykappa=cos(C_ykappa*atan(B_ykappa.*kappa_S-E_ykappa*(B_ykappa.*kappa_S-atan(B_ykappa.*kappa_S))))/G_ykappa0;















K_ygamma0=F_z*(p_Ky6+p_Ky7*df_z)*lambda_Kygamma;
S_Vygamma=F_z*(p_Vy3+p_Vy4*df_z)*gamma*lambda_Kygamma*lambda_muey*chi_2;
K_ya=p_Ky1*lambda_Fz0*F_z*sin(p_Ky4*atan(F_z/((p_Ky2+p_Ky5*gamma^2)*lambda_Fz0*F_z)))/(1+p_Ky3*gamma^2)*chi_3*lambda_Kya;
S_Vy=F_z*(p_Vy1+p_Vy2*df_z)*lambda_Vy*lambda_muey*chi_2+S_Vygamma;
S_Hy=(p_Hy1+p_Hy2*df_z)*lambda_Hy+(K_ygamma0*gamma-S_Vygamma)*chi_0/(K_ya+eps)+chi_4-1;

a_y=a+S_Hy;

D_Vykappa=mue*F_z*(r_Vy1+r_Vy2*df_z+r_Vy3*gamma)*cos(atan(r_Vy4*a))*chi_2;
S_Vykappa=D_Vykappa*sin(r_Vy5*atan(r_Vy6*kappa))*lambda_Vykappa;

C_y=p_Cy1*lambda_Cy;
D_y=mue*F_z*chi_2;
B_y=K_ya/(C_y*D_y+eps);
E_y=(p_Ey1+p_Ey2*df_z)*(1+p_Ey5*gamma^2-(p_Ey3+p_Ey4*gamma)*sign(a_y))*lambda_Ey;

F_y0=D_y*sin(C_y*atan(B_y*a_y-E_y*(B_y*a_y-atan(B_y*a_y))))+S_Vy;

F_y=G_ykappa*F_y0+S_Vykappa;

Fy=F_y;

== matlab function Model_Platform/Vehicle model/HMI_Realtime_normal_mode/HMI_Logitech1/MATLAB Function1 ==
  data: neutral input; backward_ip input; forward_ip input; forward_op output; forward_memo input; backward_memo input; backward_op output
function [forward_op, backward_op]=fcn(neutral, backward_ip, forward_ip, forward_memo, backward_memo)


if (forward_ip == 1) && (backward_ip ~= 1)
    forward_op = 1;
    backward_op = 0;
elseif (backward_ip == 1) && (forward_ip ~= 1)
    forward_op = 0;
    backward_op = 1;
elseif neutral ~= 0
    forward_op = 0;
    backward_op = 0;
else
    forward_op = forward_memo;
    backward_op = backward_memo;
end

== matlab function Model_Platform/Vehicle model/Comunication_with_visualisation_normal_mode1/Embedded MATLAB Function ==
  data: u input; y output
function y = fcn(u)
%#eml

y = typecast(u,'uint8');

== matlab function Model_Platform/Vehicle model/HMI_Realtime_normal_mode/HMI_Logitech1/MATLAB Function2 ==
  data: u input; acc output; brake output
function [acc,brake] = fcn(u)

if(u>0)
    acc=1;
    brake=1-abs(u);
else
    acc=1-abs(u);
    brake=1;
end
